simulink model "motion_example1"  (Simulink 4.00)
settings: Solver=ode45  StartTime=0.0  StopTime=3
libraries: motion x2
settings Model: LastModifiedBy=plambrec  LimitDataPoints=off  ExtModeTrigMode=oneshot  ExtModeArmWhenConnect=off

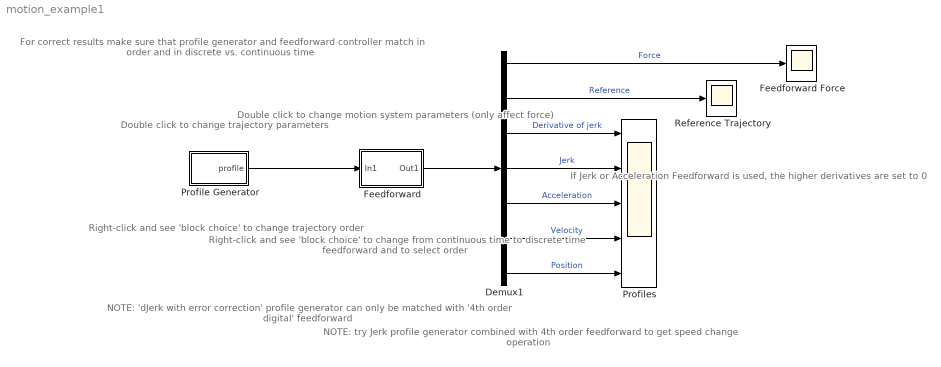
== system motion_example1 ==
  note: Double click to change
      | trajectory parameters
  note: Double click to change
      | motion system parameters
      | (only affect force)
  note: Right-click and see 'block choice'
      | to change from continuous time
      | to discrete time feedforward and
      | to select order
  note: For correct results make sure that
      | profile generator and feedforward
      | controller match in order and in
      | discrete vs. continuous time
  note: Right-click and see 'block choice'
      | to change trajectory order
  note: NOTE: 'dJerk with error correction'
      | profile generator can only be matched
      | with '4th order digital' feedforward
  note: If Jerk or Acceleration
      | Feedforward is used,
      | the higher derivatives
      | are set to 0
  note: NOTE: try Jerk profile generator
      | combined with 4th order feedforward
      | to get speed change operation
  Demux1 : Demux  Outputs=7  BusSelectionMode=off
  Feedforward : Subsystem  BlockChoice=4th order continuous
      link override 2nd order discrete: Ts=1e-1
      link override 3d order continuous: q2=0
      link override 3d order discrete: Ts=1e-1
      link override 4th order continuous: m1=20  c=6e5
      link override 4th order digital: Ts=1e-3
      link override 4th order discrete: Ts=1e-2
      settings: AttributesFormatString=%<BlockChoice>  TemplateBlock=motion/Feedforward Controllers/Feedforward  MemberBlocks=2nd order continuous,2nd order discrete,3d order continuous,3d order discrete,4th order continuous,4th order digital,4th order discrete  RTWFcnNameOpts=Auto  RTWFileNameOpts=Auto
  Feedforward Force : Scope
      settings: TimeRange=3  YMin=-150  YMax=200  SaveToWorkspace=off  SaveName=ScopeData  LimitDataPoints=on  MaxDataPoints=50000
  Profile Generator : Subsystem  BlockChoice=Derivative of Jerk
      link override Acceleration: Ts=1e-1  a=5
      link override Derivative of Jerk: Ts=1e-2
      link override Jerk: Ts=0
      link override dJerk with error correction: Ts=1e-3
      settings: AttributesFormatString=%<BlockChoice>  TemplateBlock=motion/Profile Generators/Profile Generator  MemberBlocks=Acceleration,Derivative of Jerk,Jerk,dJerk with error correction  RTWFcnNameOpts=Auto  RTWFileNameOpts=Auto
  Profiles : Scope  NumInputPorts=5
      settings: TimeRange=3  YMin=-1000~-100~-5~0~-0.5  YMax=1000~100~10~1.5~1.5  SaveToWorkspace=off  SaveName=ScopeData2  LimitDataPoints=on  MaxDataPoints=50000
  Reference Trajectory : Scope
      settings: TimeRange=3  YMin=-0.2  YMax=1.2  SaveToWorkspace=off  LimitDataPoints=on  MaxDataPoints=50000
  wires:
  Feedforward/1(Out1) -> Demux1/1
  Demux1/1 -> Feedforward Force/1  "Force"
  Demux1/2 -> Reference Trajectory/1  "Reference"
  Demux1/3 -> Profiles/1  "Derivative of jerk"
  Demux1/4 -> Profiles/2  "Jerk"
  Demux1/5 -> Profiles/3  "Acceleration"
  Demux1/6 -> Profiles/4  "Velocity"
  Demux1/7 -> Profiles/5  "Position"
  Profile Generator/1(profile) -> Feedforward/1(In1)

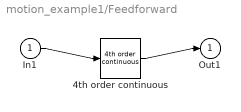
== system motion_example1/Feedforward ==
  In1 : Inport  Port=1
  4th order continuous : motion/Feedforward Controllers/4th order continuous  m1=20  m2=10  k1=10  k2=10  c=6e5  k12=500
  Out1 : Outport  Port=1
  wires:
  In1/1 -> 4th order continuous/1
  4th order continuous/1 -> Out1/1

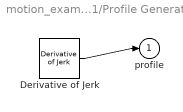
== system motion_example1/Profile Generator ==
  Derivative of Jerk : motion/Profile Generators/Derivative of Jerk  AncestorBlock=library/Derivative of jerk profile generator  t0=.3  x=1  v=1  a=5  j=50  d=1000  Ts=1e-2
  profile : Outport  Port=1
  wires:
  Derivative of Jerk/1 -> profile/1
